simulink model "z2_5_simulacija"  (R2018a)
settings: Solver=VariableStepAuto  StartTime=0.0  StopTime=10.0  RelTol=1e-3
values from neighbouring files (symbols this model uses):
  I = ((10+P2)^2)/4 + 100    (= 136)    [z2_5.m]
  P1 = -11    [z2_5.m]
  P2 = 2    [z2_5.m]
settings Model: Creator=djoco  LastModifiedBy=djoco

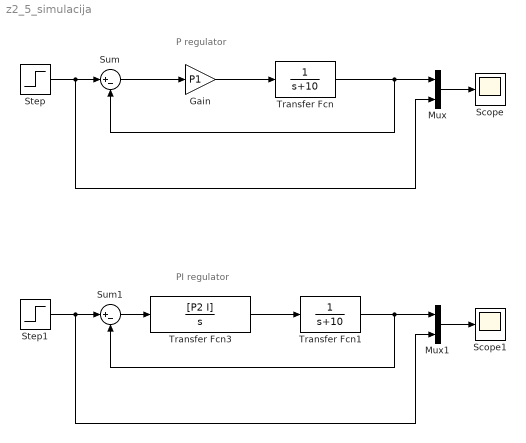
== system z2_5_simulacija ==
  note: P regulator
  note: PI regulator
  Gain : Gain  Gain=P1
  Mux : Mux  Inputs=2
  Mux1 : Mux  Inputs=2
  Scope : Scope
  Scope1 : Scope
  Step : Step  SampleTime=0
  Step1 : Step  SampleTime=0
  Sum : Sum  Inputs=|+-
  Sum1 : Sum  Inputs=|+-
  Transfer Fcn : TransferFcn  Denominator=[1 10]
  Transfer Fcn1 : TransferFcn  Denominator=[1 10]
  Transfer Fcn3 : TransferFcn  Numerator=[P2 I]  Denominator=[1 0]
  wires:
  Transfer Fcn/1 -> Sum/2, Mux/1
  Step/1 -> Mux/2, Sum/1
  Mux/1 -> Scope/1
  Mux1/1 -> Scope1/1
  Step1/1 -> Mux1/2, Sum1/1
  Transfer Fcn1/1 -> Sum1/2, Mux1/1
  Gain/1 -> Transfer Fcn/1
  Sum/1 -> Gain/1
  Transfer Fcn3/1 -> Transfer Fcn1/1
  Sum1/1 -> Transfer Fcn3/1
